simulink model "Example"  (R2023b)
settings: Solver=VariableStepAuto  StartTime=0.0  StopTime=50  RelTol=1e-3
values from neighbouring files (symbols this model uses):
  T = 0.1    [programa.m]
libraries: fuzblock x1
settings Model: Creator=usuario  LastModifiedBy=usuario
settings DataIOCC: ReturnWorkspaceOutputs=off

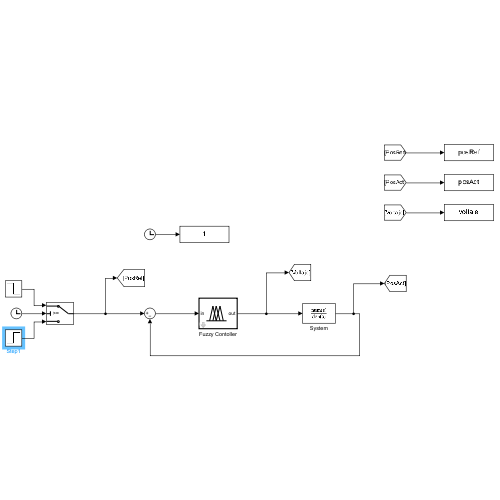
[thumbnail: Simulink's stored preview of the top-level diagram]
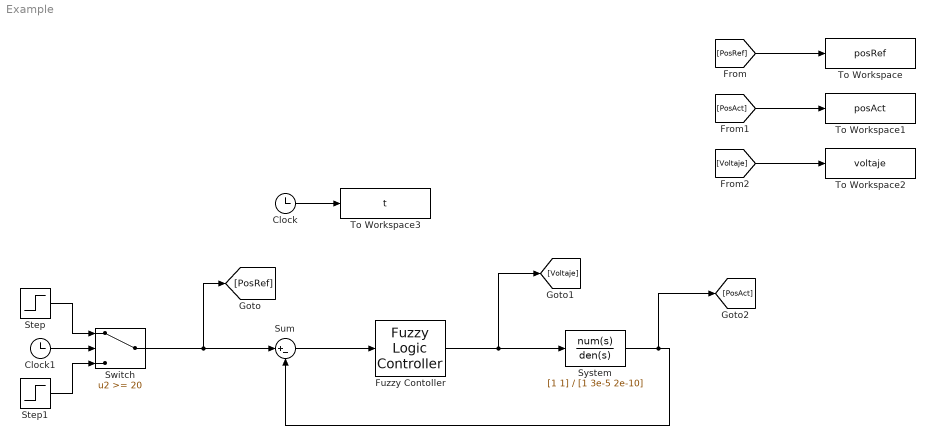
== system Example ==
  Clock : Clock
  Clock1 : Clock
  Fuzzy Contoller : fuzblock/Fuzzy Logic  Controller  FIS=example  OutputSampleNumber=101  DataType=double  FuzzifiedInputs=off  RuleFiringStrengths=off  RuleOutputs=off  AggregatedOutputs=off  SimulateUsing=Interpreted execution  OutOfRangeInputValueMessage=warning  NoRuleFiredMessage=warning  EmptyOutputFuzzySetMessage=warning
  Step : Step  Time=20  After=-5  SampleTime=0
  Step1 : Step  Time=2  After=5  SampleTime=0
  Sum : Sum  Inputs=|+-
  Switch : Switch  Threshold=20  SaturateOnIntegerOverflow=off  InputSameDT=off
  System : TransferFcn  Numerator=[1 1]  Denominator=[1 3e-5 2e-10]
  To Workspace : ToWorkspace  VariableName=posRef  SampleTime=T
  To Workspace1 : ToWorkspace  VariableName=posAct  SampleTime=T
  To Workspace2 : ToWorkspace  VariableName=voltaje  SampleTime=T
  To Workspace3 : ToWorkspace  VariableName=t  SampleTime=T
  wires:
  Switch/1 -> [PosRef], Sum/1
  System/1 -> [PosAct], Sum/2
  Sum/1 -> Fuzzy Contoller/1
  Fuzzy Contoller/1 -> [Voltaje], System/1
  Clock/1 -> To Workspace3/1
  [PosRef] -> To Workspace/1
  [PosAct] -> To Workspace1/1
  [Voltaje] -> To Workspace2/1
  Clock1/1 -> Switch/2
  Step1/1 -> Switch/3
  Step/1 -> Switch/1
